simulink model "example_Storage_type0"  (R2018b)
settings: Solver=ode45  StartTime=0.0  StopTime=3*3600-2  MaxStep=300  RelTol=1e-3  EnableMultiTasking=on
undefined symbols (not defined in the file): path_carnot
libraries: carnot x5, simulink x1
settings Model: Creator=drhf  LastModifiedBy=P41573
settings DataIOCC: LimitDataPoints=on  SaveFormat=Array
settings OptimizationCC: ExpressionDepthLimit=2147483647  LifeSpan=inf
settings DebuggingCC: UnderspecifiedInitializationDetection=Classic  MergeDetectMultiDrivingBlocksExec=none  SolverPrmCheckMsg=warning  StateNameClashWarn=warning  SFUnexpectedBacktrackingDiag=warning  SFNoUnconditionalDefaultTransitionDiag=warning  SFExecutionAtInitializationDiag=none
settings HardwareCC: ProdBitPerPointer=32  ProdBitPerSizeT=32  ProdBitPerPtrDiffT=32  ProdLargestAtomicFloat=None  ProdIntDivRoundTo=Undefined  ProdEndianess=Unspecified  ProdWordSize=32  ProdHWDeviceType=32-bit Generic
settings ModelReferenceCC: PropagateSignalLabelsOutOfModel=off
settings SFSimCC: SimUseLocalCustomCode=off
settings RTWCC: RTWUseLocalCustomCode=off
settings CodeAppCC: StateflowObjectComments=on
settings GRTTargetCC: TargetLangStandard=C89/C90 (ANSI)  GeneratePreprocessorConditionals=Disable all  CombineOutputUpdateFcns=off  GRTInterface=on
settings ConfigComp: CovMetricSettings=dw  CovHtmlReporting=on  CovSaveCumulativeToWorkspaceVar=on  CovSaveSingleToWorkspaceVar=on  CovExternalEMLEnable=off

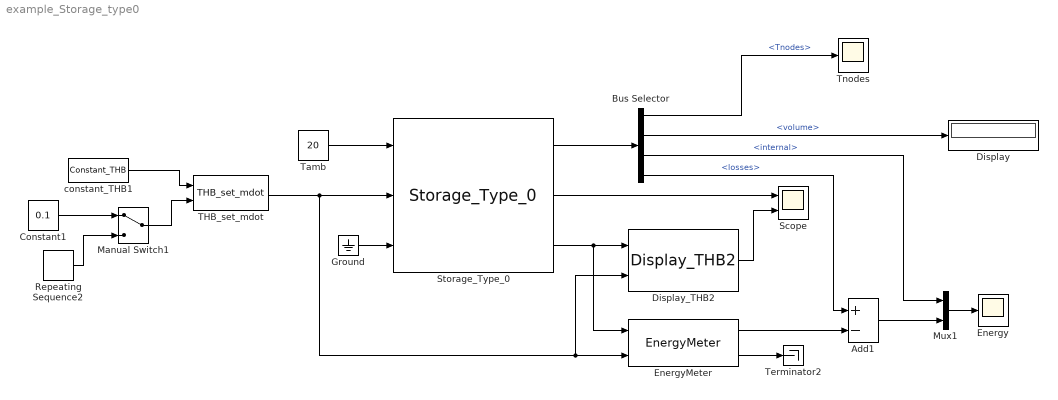
== system example_Storage_type0 ==
  Add1 : Sum  Inputs=+-
  Bus Selector : BusSelector  OutputSignals=Tnodes,volume,energy.internal,energy.losses
  Constant1 : Constant  Value=0.1
  Display : Display
  Display_THB2 : carnot/Outputs/Display_THB2  t=off  m=on  p=off  id=off  mix=off  d=off
      settings: SourceProductName=Carnot
  Energy : Scope
  EnergyMeter : carnot/Control/EnergyMeter
      settings: SourceProductName=Carnot
  Ground : Ground
  Manual Switch1 : ManualSwitch
  Mux1 : Mux  Inputs=2
  Repeating Sequence2 : simulink/Sources/Repeating Sequence  rep_seq_t=[ 0 3600 3600+eps(3600) 7200 7200+eps(7200) 10440 10440+eps(10440) 11160]  rep_seq_y=[ 0.12 0.12 0.15+0*eps(3600) 0.15 0.1+0*eps(7200) 0.1 0+0*eps(10440) 0]
  Scope : Scope  NumInputPorts=2
  Storage_Type_0 : carnot/Storage/Thermal/Storage_Type_0  t0=[10:5:55]  hgt=1.5279  stgtype=0  mpts=[1 2 3 4 5 6 7 8 9 10]  tini=[10 15 20 25 30 35 40 45 50 55]  PathName=fullfile(path_carnot('libsl'),'Storage','Thermal','Storage_Type_0','parameter_set')  FileName='StorageTyp0_300_L.mat'  userPath=off  userParam=off  uwall=1  ubot=1  utop=1  axcond=1  volume=0.3  dia=0.5  standing=standing cylinder  nodes=10  mpoints=10  Tsensor=0.5  pipe1inlet=1  pipe1outlet=0  pipe1dia=0.03  heater1start=0.2  heater1end=0.25
      settings: SourceProductName=Carnot
  THB_set_mdot : carnot/Source/Simple/THB_set_mdot
      settings: SourceProductName=Carnot
  Tamb : Constant  Value=20
  Terminator2 : Terminator
  Tnodes : Scope
  constant_THB1 : carnot/Source/Simple/Constant_THB  t=55  mdot=0*100/3600  p=1e5  mID=Full Pressure Drop with Static Height  fluid=Water  mix=0  mix2=0  mix3=0  dia=0.02  hgt=0
      settings: SourceProductName=Carnot
  wires:
  Bus Selector/3 -> Mux1/1  "<internal>"
  Tamb/1 -> Storage_Type_0/1
  THB_set_mdot/1 -> Display_THB2/2, EnergyMeter/2, Storage_Type_0/2
  Storage_Type_0/1 -> Bus Selector/1
  Storage_Type_0/2 -> Scope/1
  Storage_Type_0/3 -> EnergyMeter/1, Display_THB2/1
  Display_THB2/1 -> Scope/2
  Mux1/1 -> Energy/1
  constant_THB1/1 -> THB_set_mdot/1
  Manual Switch1/1 -> THB_set_mdot/2
  Constant1/1 -> Manual Switch1/1
  Repeating Sequence2/1 -> Manual Switch1/2
  EnergyMeter/2 -> Terminator2/1
  Add1/1 -> Mux1/2
  EnergyMeter/1 -> Add1/2
  Bus Selector/4 -> Add1/1  "<losses>"
  Bus Selector/2 -> Display/1  "<volume>"
  Bus Selector/1 -> Tnodes/1  "<Tnodes>"
  Ground/1 -> Storage_Type_0/3
